simulink model "model1"  (R2024a)
settings: Solver=ode23t  StartTime=0.0  StopTime=finalatt{end,1}  MaxStep=0.1  RelTol=1e-3
undefined symbols (not defined in the file): finalatt, FrontAxle, FrontGear, MassWheel, NewData, RadiusWheel, RearAxle, RearGear, SlipAngle, TrackData, VehicleMass
libraries: fl_lib x16, batt_lib x13, nesl_utility x11, sdl_lib x7, ee_lib x2, simulink x1
(part 2 of 2)

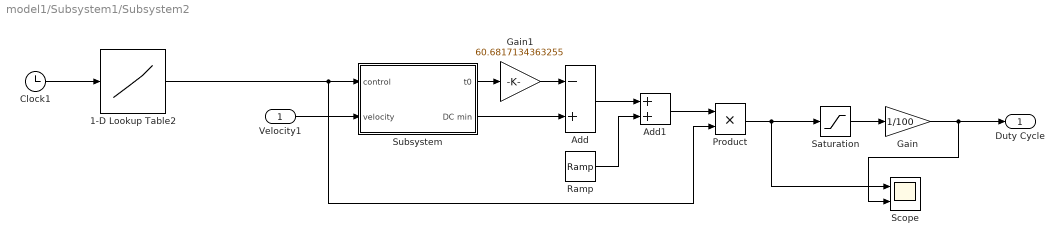
== system model1/Subsystem1/Subsystem2 ==
  Velocity1 : Inport
  1-D Lookup Table2 : Lookup_n-D  NumberOfTableDimensions=1  BreakpointsForDimension1=finalatt{:,1}  Table=finalatt{:,3}  InterpMethod=Flat  InternalRulePriority=Speed  RndMeth=Simplest
  Add : Sum  Inputs=-+
  Add1 : Sum
  Clock1 : Clock
      settings: Decimation=1000
  Gain : Gain  Gain=1/100
  Gain1 : Gain  Gain=60.6817134363255
  Product : Product
  Ramp : simulink/Sources/Ramp  slope=60.6817134363255  start=0  InitialOutput=0
  Saturation : Saturate  UpperLimit=95  LowerLimit=0
  Scope : Scope  NumInputPorts=2
  Subsystem : Subsystem
  Duty Cycle : Outport
  wires:
  Clock1/1 -> 1-D Lookup Table2/1
  Product/1 -> Scope/1, Saturation/1
  Ramp/1 -> Add1/2
  Add1/1 -> Product/1
  Gain1/1 -> Add/1
  Velocity1/1 -> Subsystem/2(velocity)
  Add/1 -> Add1/1
  1-D Lookup Table2/1 -> Product/2, Subsystem/1(control)
  Subsystem/2(DC min) -> Add/2
  Subsystem/1(t0) -> Gain1/1
  Gain/1 -> Scope/2, Duty Cycle/1
  Saturation/1 -> Gain/1

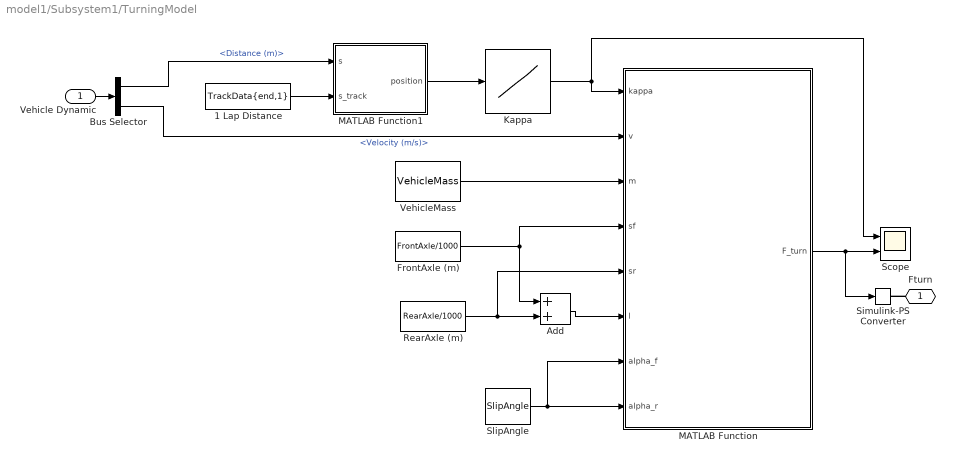
== system model1/Subsystem1/TurningModel ==
  Vehicle Dynamic : Inport
  1 Lap Distance : Constant  Value=TrackData{end,1}
  Add : Sum
  Bus Selector : BusSelector  OutputSignals=Distance (m),Velocity (m/s)
  FrontAxle (m) : Constant  Value=FrontAxle/1000
  Kappa : Lookup_n-D  NumberOfTableDimensions=1  BreakpointsForDimension1=TrackData{:,1}  Table=TrackData{:,4}  InternalRulePriority=Speed  RndMeth=Simplest
  MATLAB Function : MATLAB Function  TreatAsAtomicUnit=on
  MATLAB Function1 : MATLAB Function  TreatAsAtomicUnit=on
  RearAxle (m) : Constant  Value=RearAxle/1000
  Scope : Scope  NumInputPorts=2
  Simulink-PS Converter : nesl_utility/Simulink-PS Converter  PhysicalDomain=network_engine_domain  SubClassName=ps_input  LeftPortType=input  RightPortType=output  PseudoPeriodic=off  Frequencies=[]  NoiseDistribution=none  NoiseParameters=[]  Unit=N  AffineConversion=off  FilteringAndDerivatives=provide  SimscapeFilterOrder=1  InputFilterTimeConstant=0.001  UdotUserProvided=0
  SlipAngle : Constant  Value=SlipAngle
  VehicleMass : Constant  Value=VehicleMass
  Fturn : PMIOPort  Side=Left
  wires:
  VehicleMass/1 -> MATLAB Function/3(m)
  1 Lap Distance/1 -> MATLAB Function1/2(s_track)
  Kappa/1 -> Scope/1, MATLAB Function/1(kappa)
  RearAxle (m)/1 -> MATLAB Function/5(sr), Add/2
  FrontAxle (m)/1 -> MATLAB Function/4(sf), Add/1
  Bus Selector/1 -> MATLAB Function1/1(s)  "<Distance (m)>"
  MATLAB Function1/1(position) -> Kappa/1
  SlipAngle/1 -> MATLAB Function/7(alpha_f), MATLAB Function/8(alpha_r)
  MATLAB Function/1(F_turn) -> Simulink-PS Converter/1, Scope/2
  Vehicle Dynamic/1 -> Bus Selector/1
  Bus Selector/2 -> MATLAB Function/2(v)  "<Velocity (m/s)>"
  Add/1 -> MATLAB Function/6(l)
  connections:
  Fturn/RConn1 -- Simulink-PS Converter/RConn1

== system model1/Subsystem1/VehicleModel ==
  Ideal Force Source : fl_lib/Mechanical/Mechanical Sources/Ideal Force Source
  Mechanical Translational Reference : fl_lib/Mechanical/Translational Elements/Mechanical Translational Reference
  PS Gain : fl_lib/Physical Signals/Functions/PS Gain  gain=0.5
  PS Terminator3 : fl_lib/Physical Signals/Sinks/PS Terminator
  TireModel : Subsystem
      settings: PortSchema="{\"entries\":[{\"content\":{\"sides\":[{\"content\":{\"connectorIds\":[\"LConn1\",\"LConn2\"]},\"type\":\"ConnectorPlacement.EquallySpacedRectSide\",\"uuid\":\"ad88246c-79e4-4500-822e-5fea39c5896c\"},{\"content\":{\"connectorIds\":[\"Out1\"],\"side\":\"RIGHT\"},\"type\":\"ConnectorPlacement.EquallySpacedRectSide\",\"uuid\":\"913d52ca-54a5-4560-b3df-e1f57975974a\"},{\"content\":{\"connectorIds\":[\"LConn3\",\"LConn4\",\"LConn5\"],\"side\":\"TOP\"},\"type\":\"ConnectorPlacement.EquallySpacedRectSide\",\"uuid\":\"5900099e-62c2-49ce-8123-88bd27d24a29\"}]},\"type\":\"ConnectorPlacement.EquallySpacedConnector\",\"uuid\":\"881a997e-2d63-4bf2-b975-40b530568104\"}],\"packageUris\":[\"http://schema.mathworks.com/mf0/Connector/R2020b\"],\"version\":\"1.0\"}"
  Vehicle Body : sdl_lib/Tires & Vehicles/Vehicle Body  mass=VehicleMass kg  n_w=1  x_f=FrontAxle mm  x_r=RearAxle mm  y_c=GroundClearance mm  mass_var=simscape.enum.onoff.off  g=9.81 m/s^2  liftoff_warning=simscape.enum.onoff.off  area=FrontArea m^2  Cd=CD  rho=1.18 kg/m^3  model_pitch=simscape.enum.onoff.off  inertia=4000 kg*m^2  suspension_model=sdl.enum.linearTLU.linear  k_f=1e4 N/m  b_f=1e4 N*s/m  k_r=1e4 N/m  b_r=1e4 N*s/m  k_f_TLU=[-2000, -1000, 0, 1000, 2000] N  x_f_TLU=[-.4, -.2, 0, .2, .4] m  b_f_TLU=[-200, -100, 0, 100, 200] N  v_f_TLU=[-4, -2, 0, 2, 4] m/s  k_r_TLU=[-2000, -1000, 0, 1000, 2000] N  x_r_TLU=[-.4, -.2, 0, .2, .4] m  b_r_TLU=[-200, -100, 0, 100, 200] N  v_r_TLU=[-4, -2, 0, 2, 4] m/s  interp_method=simscape.enum.interpolation.linear  extrap_method=simscape.enum.extrapolation.linear  model_hardstop=simscape.enum.onoff.off  upper_bound_f=.25 m  lower_bound_f=-.25 m  stop_k_f=1e6 N/m  stop_b_f=150 N*s/m  upper_bound_r=.25 m  lower_bound_r=-.25 m  stop_k_r=1e6 N/m  stop_b_r=150 N*s/m  initial_pitch=0 rad  initial_pitch_rate=0 rad/s  v_specify=off  v_priority=High  v=0 m/s  v_nominal_specify=off  v_nominal_value=1  v_nominal_unit=m/s
  FromClutch : PMIOPort  Side=Left
  Fturn : PMIOPort  Port=2  Side=Right
  VehicleDynamic : Outport
  wires:
  TireModel/1(VehicleDynamic) -> VehicleDynamic/1
  connections:
  TireModel/LConn2 -- FromClutch/RConn1
  Vehicle Body/RConn1 -- TireModel/LConn3
  Ideal Force Source/LConn1 -- Mechanical Translational Reference/LConn1
  Ideal Force Source/RConn2 -- TireModel/LConn1 -- Vehicle Body/LConn1
  Fturn/RConn1 -- Ideal Force Source/RConn1
  PS Gain/LConn1 -- Vehicle Body/RConn2
  PS Gain/RConn1 -- TireModel/LConn4
  PS Terminator3/LConn1 -- Vehicle Body/LConn2

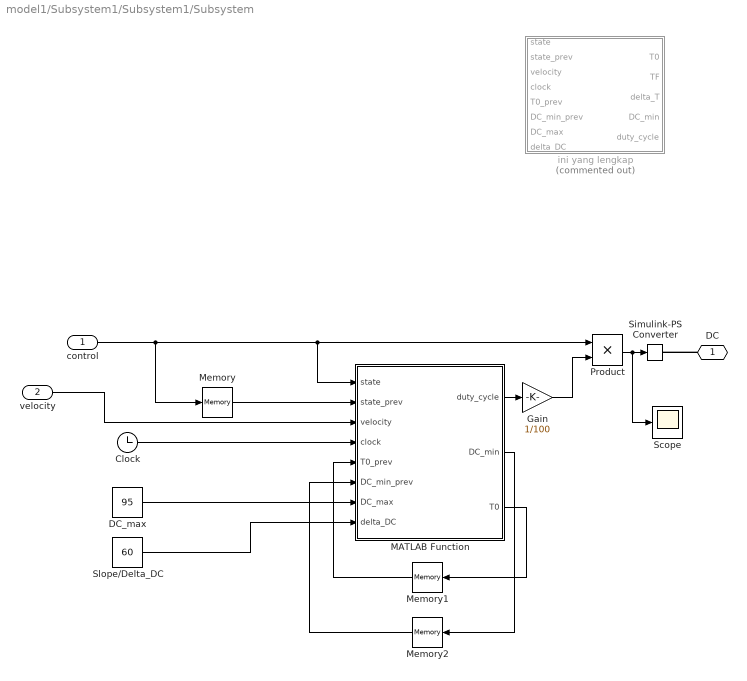
== system model1/Subsystem1/Subsystem1/Subsystem ==
  control : Inport
  velocity : Inport  Port=2
  Clock : Clock
  DC_max : Constant  Value=95
  Gain : Gain  Gain=1/100
  MATLAB Function : MATLAB Function  TreatAsAtomicUnit=on
  Memory : Memory
  Memory1 : Memory
  Memory2 : Memory
  Product : Product
  Scope : Scope
  Simulink-PS Converter : nesl_utility/Simulink-PS Converter  PhysicalDomain=network_engine_domain  SubClassName=ps_input  LeftPortType=input  RightPortType=output  PseudoPeriodic=off  Frequencies=[]  NoiseDistribution=none  NoiseParameters=[]  Unit=1  AffineConversion=off  FilteringAndDerivatives=provide  SimscapeFilterOrder=1  InputFilterTimeConstant=0.001  UdotUserProvided=0
  Slope/Delta_DC : Constant  Value=60
  ini yang lengkap : MATLAB Function  Commented=on  TreatAsAtomicUnit=on
  DC : PMIOPort  Side=Right
  wires:
  Clock/1 -> MATLAB Function/4(clock)
  control/1 -> Memory/1, MATLAB Function/1(state), Product/1
  Memory/1 -> MATLAB Function/2(state_prev)
  velocity/1 -> MATLAB Function/3(velocity)
  DC_max/1 -> MATLAB Function/7(DC_max)
  Slope/Delta_DC/1 -> MATLAB Function/8(delta_DC)
  Product/1 -> Simulink-PS Converter/1, Scope/1
  Memory1/1 -> MATLAB Function/5(T0_prev)
  MATLAB Function/3(T0) -> Memory1/1
  MATLAB Function/2(DC_min) -> Memory2/1
  Memory2/1 -> MATLAB Function/6(DC_min_prev)
  MATLAB Function/1(duty_cycle) -> Gain/1
  Gain/1 -> Product/2
  connections:
  DC/RConn1 -- Simulink-PS Converter/RConn1

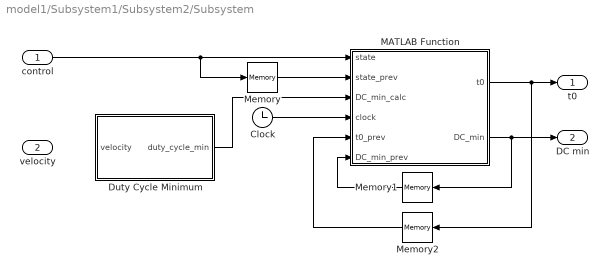
== system model1/Subsystem1/Subsystem2/Subsystem ==
  control : Inport
  velocity : Inport  Port=2
  Clock : Clock
  Duty Cycle Minimum : MATLAB Function  TreatAsAtomicUnit=on
  MATLAB Function : MATLAB Function  TreatAsAtomicUnit=on
  Memory : Memory
  Memory1 : Memory
  Memory2 : Memory
  t0 : Outport
  DC min : Outport  Port=2
  wires:
  MATLAB Function/1(t0) -> Memory2/1, t0/1
  Clock/1 -> MATLAB Function/4(clock)
  control/1 -> Memory/1, MATLAB Function/1(state)
  Memory/1 -> MATLAB Function/2(state_prev)
  MATLAB Function/2(DC_min) -> DC min/1, Memory1/1
  Memory1/1 -> MATLAB Function/6(DC_min_prev)
  Memory2/1 -> MATLAB Function/5(t0_prev)
  Duty Cycle Minimum/1(duty_cycle_min) -> MATLAB Function/3(DC_min_calc)

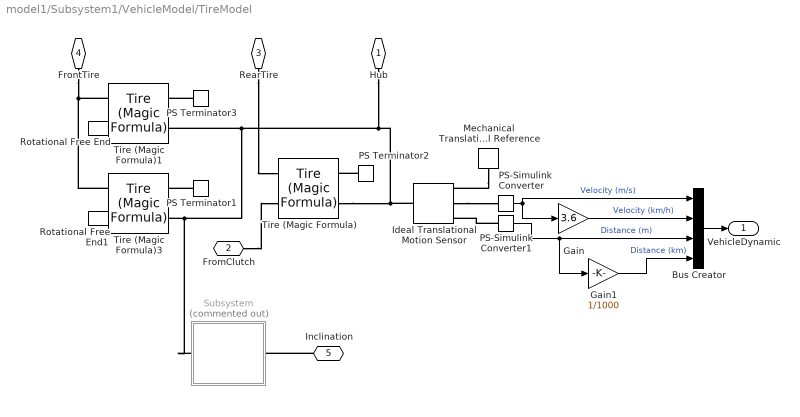
== system model1/Subsystem1/VehicleModel/TireModel ==
  Bus Creator : BusCreator  Inputs=4
  Gain : Gain  Gain=3.6
  Gain1 : Gain  Gain=1/1000
  Ideal Translational Motion Sensor : fl_lib/Mechanical/Mechanical Sensors/Ideal Translational Motion Sensor  reference=foundation.enum.MeasurementReference.difference  acceleration_port=false  velocity_port=true  position_port=true  offset=0 m
  Mechanical Translational Reference : fl_lib/Mechanical/Translational Elements/Mechanical Translational Reference
  PS Terminator1 : fl_lib/Physical Signals/Sinks/PS Terminator
  PS Terminator2 : fl_lib/Physical Signals/Sinks/PS Terminator
  PS Terminator3 : fl_lib/Physical Signals/Sinks/PS Terminator
  PS-Simulink Converter : nesl_utility/PS-Simulink Converter  PhysicalDomain=network_engine_domain  SubClassName=ps_output  LeftPortType=input  RightPortType=output  PseudoPeriodic=off  Frequencies=[]  VectorFormat=1-D array  Unit=m/s  AffineConversion=off
  PS-Simulink Converter1 : nesl_utility/PS-Simulink Converter  PhysicalDomain=network_engine_domain  SubClassName=ps_output  LeftPortType=input  RightPortType=output  PseudoPeriodic=off  Frequencies=[]  VectorFormat=1-D array  Unit=m  AffineConversion=off
  Rotational Free End : fl_lib/Mechanical/Rotational Elements/Rotational Free End  w_specify=off  w_priority=None  w=0 rad/s  w_nominal_specify=off  w_nominal_value=1  w_nominal_unit=rad/s
  Rotational Free End1 : fl_lib/Mechanical/Rotational Elements/Rotational Free End  w_specify=off  w_priority=None  w=0 rad/s  w_nominal_specify=off  w_nominal_value=1  w_nominal_unit=rad/s
  Subsystem : Subsystem  Commented=on
  Tire (Magic Formula) : sdl_lib/Tires & Vehicles/Tire (Magic Formula)  parameterization=sdl.enum.magic_tire_model.peak  F_z1=3000 N  F_x1=3500 N  kappa1=10  B_m=10  C_m=1.9  D_m=1  E_m=0.97  fz0=4000 N  p_Cx=1.685  p_Dx=[1.21, -.037]  p_Ex=[.344, .095, -.02, 0]  p_Kx=[21.51, -.163, .245]  p_Hx=[-.002, .002]  p_Vx=[0, 0]  rolling_radius_model=sdl.enum.RollingRadiusParameterization.Constant  r_e=RadiusWheel m  r_0=0.3 m  breff=8.39  dreff=0.26  freff=0.074  q_re0=0.99  q_v1=0.008  longvl=17 m/s  cz=5e5 N/m  model_resistance=true  resistance_model=sdl.enum.rollingResistanceParameterization.constant  coeff=CRR  p_tire=250e3 Pa  alpha=-0.003  beta=0.97  coeff_a=84e-4  coeff_b=6.2e-4 s/m  coeff_c=1.6e-4 s^2/m^2  p_tire0=240e3 Pa  fz0_resistance=4000 N  vH0=16 m/s  q_Sy=[.0082, 0, .0014, .001, 0, 0, 1.08, -.5]  v_thr=0.001 m/s  enable_scaling_coefficients=false  lfzO=1  lcx=1  lmux=1  lex=1  lkx=1  lhx=1  lvx=1  lmy=1  model_compliance=sdl.enum.compliance.off  stiffness=1e6 N/m  damping=1000 N*s/m  model_inertia=sdl.enum.model_inertia.on  inertia=MassWheel*RadiusWheel^2 kg*m^2  initial_velocity=0 rad/s  vxlow=1 m/s  v_tr_thr=0.1 m/s  kpumin=-1.5  kpumax=1.5
  Tire (Magic Formula)1 : sdl_lib/Tires & Vehicles/Tire (Magic Formula)  parameterization=sdl.enum.magic_tire_model.peak  F_z1=3000 N  F_x1=3500 N  kappa1=10  B_m=10  C_m=1.9  D_m=1  E_m=0.97  fz0=4000 N  p_Cx=1.685  p_Dx=[1.21, -.037]  p_Ex=[.344, .095, -.02, 0]  p_Kx=[21.51, -.163, .245]  p_Hx=[-.002, .002]  p_Vx=[0, 0]  rolling_radius_model=sdl.enum.RollingRadiusParameterization.Constant  r_e=RadiusWheel m  r_0=0.3 m  breff=8.39  dreff=0.26  freff=0.074  q_re0=0.99  q_v1=0.008  longvl=17 m/s  cz=5e5 N/m  model_resistance=true  resistance_model=sdl.enum.rollingResistanceParameterization.constant  coeff=CRR  p_tire=250e3 Pa  alpha=-0.003  beta=0.97  coeff_a=84e-4  coeff_b=6.2e-4 s/m  coeff_c=1.6e-4 s^2/m^2  p_tire0=240e3 Pa  fz0_resistance=4000 N  vH0=16 m/s  q_Sy=[.0082, 0, .0014, .001, 0, 0, 1.08, -.5]  v_thr=0.001 m/s  enable_scaling_coefficients=false  lfzO=1  lcx=1  lmux=1  lex=1  lkx=1  lhx=1  lvx=1  lmy=1  model_compliance=sdl.enum.compliance.off  stiffness=1e6 N/m  damping=1000 N*s/m  model_inertia=sdl.enum.model_inertia.on  inertia=MassWheel*RadiusWheel^2 kg*m^2  initial_velocity=0 rad/s  vxlow=1 m/s  v_tr_thr=0.1 m/s  kpumin=-1.5  kpumax=1.5
  Tire (Magic Formula)3 : sdl_lib/Tires & Vehicles/Tire (Magic Formula)  parameterization=sdl.enum.magic_tire_model.peak  F_z1=3000 N  F_x1=3500 N  kappa1=10  B_m=10  C_m=1.9  D_m=1  E_m=0.97  fz0=4000 N  p_Cx=1.685  p_Dx=[1.21, -.037]  p_Ex=[.344, .095, -.02, 0]  p_Kx=[21.51, -.163, .245]  p_Hx=[-.002, .002]  p_Vx=[0, 0]  rolling_radius_model=sdl.enum.RollingRadiusParameterization.Constant  r_e=RadiusWheel m  r_0=0.3 m  breff=8.39  dreff=0.26  freff=0.074  q_re0=0.99  q_v1=0.008  longvl=17 m/s  cz=5e5 N/m  model_resistance=true  resistance_model=sdl.enum.rollingResistanceParameterization.constant  coeff=CRR  p_tire=250e3 Pa  alpha=-0.003  beta=0.97  coeff_a=84e-4  coeff_b=6.2e-4 s/m  coeff_c=1.6e-4 s^2/m^2  p_tire0=240e3 Pa  fz0_resistance=4000 N  vH0=16 m/s  q_Sy=[.0082, 0, .0014, .001, 0, 0, 1.08, -.5]  v_thr=0.001 m/s  enable_scaling_coefficients=false  lfzO=1  lcx=1  lmux=1  lex=1  lkx=1  lhx=1  lvx=1  lmy=1  model_compliance=sdl.enum.compliance.off  stiffness=1e6 N/m  damping=1000 N*s/m  model_inertia=sdl.enum.model_inertia.on  inertia=MassWheel*RadiusWheel^2 kg*m^2  initial_velocity=0 rad/s  vxlow=1 m/s  v_tr_thr=0.1 m/s  kpumin=-1.5  kpumax=1.5
  Hub : PMIOPort  Side=Left
  FromClutch : PMIOPort  Port=2  Side=Left
  RearTire : PMIOPort  Port=3  Side=Left
  FrontTire : PMIOPort  Port=4  Side=Left
  Inclination : PMIOPort  Port=5  Side=Left
  VehicleDynamic : Outport
  wires:
  PS-Simulink Converter1/1 -> Gain1/1, Bus Creator/3  "Distance (m)"
  PS-Simulink Converter/1 -> Bus Creator/1, Gain/1  "Velocity (m/s)"
  Gain/1 -> Bus Creator/2  "Velocity (km/h)"
  Bus Creator/1 -> VehicleDynamic/1
  Gain1/1 -> Bus Creator/4  "Distance (km)"
  connections:
  PS Terminator3/LConn1 -- Tire (Magic Formula)1/RConn1
  FrontTire/RConn1 -- Tire (Magic Formula)1/LConn1 -- Tire (Magic Formula)3/LConn1
  Tire (Magic Formula)/RConn2 -- Ideal Translational Motion Sensor/LConn1 -- Hub/RConn1 -- Tire (Magic Formula)1/RConn2 -- Subsystem/RConn1 -- Tire (Magic Formula)3/RConn2
  Tire (Magic Formula)1/LConn2 -- Rotational Free End/LConn1
  Tire (Magic Formula)3/LConn2 -- Rotational Free End1/LConn1
  PS Terminator1/LConn1 -- Tire (Magic Formula)3/RConn1
  RearTire/RConn1 -- Tire (Magic Formula)/LConn1
  PS Terminator2/LConn1 -- Tire (Magic Formula)/RConn1
  FromClutch/RConn1 -- Tire (Magic Formula)/LConn2
  Mechanical Translational Reference/LConn1 -- Ideal Translational Motion Sensor/RConn1
  PS-Simulink Converter1/LConn1 -- Ideal Translational Motion Sensor/RConn3
  Ideal Translational Motion Sensor/RConn2 -- PS-Simulink Converter/LConn1
  Inclination/RConn1 -- Subsystem/LConn1

== system model1/Subsystem1/VehicleModel/TireModel/Subsystem ==
  PS-Simulink Converter2 : nesl_utility/PS-Simulink Converter  Commented=on  PhysicalDomain=network_engine_domain  SubClassName=ps_output  LeftPortType=input  RightPortType=output  PseudoPeriodic=off  Frequencies=[]  VectorFormat=inherit  Unit=inherit  AffineConversion=off
  Road Profile : sdl_lib/Tires & Vehicles/Road Profile  Commented=on  x_f=FrontAxle mm  x_r=RearAxle mm  x_height_vector=TrackData{:,1} m  height_vector=TrackData{:,6} m  friction_output=sdl.enum.tire_friction_model.none  x_friction_vector=[-10, 2, 2.1, 6, 6.1, 10] m  MF_M_matrix=[10, 2, 1, 1; 10, 2, 1, 1; 8, 3, 1, 1; 8, 3, 1, 1; 9, 4, 1, 1; 9, 4, 1, 1]  MR_M_matrix=[10, 2, 1, 1; 10, 2, 1, 1; 8, 3, 1, 1; 8, 3, 1, 1; 9, 4, 1, 1; 9, 4, 1, 1]  MF_F_matrix=[.9, .7; .9, .7; .7, .5; .7, .5; .8, .6; .8, .6]  MR_F_matrix=[.9, .7; .9, .7; .7, .5; .7, .5; .8, .6; .8, .6]  x_specify=off  x_priority=High  x=0 m  x_nominal_specify=off  x_nominal_value=1  x_nominal_unit=m
      settings: InternalSimscapePortConfiguration="{\"Bottom\":[],\"Left\":[],\"Right\":[{\"id\":\"H\",\"label\":\"H\",\"type\":\"foundation.mechanical.translational.translational\"},{\"id\":\"beta\",\"label\":\"beta\",\"type\":\"output\"}],\"Top\":[]}"
  Scope : Scope  Commented=on
  Conn1 : PMIOPort  Side=Right
  Inclination : PMIOPort  Port=2  Side=Left
  wires:
  PS-Simulink Converter2/1 -> Scope/1
  connections:
  PS-Simulink Converter2/LConn1 -- Inclination/RConn1 -- Road Profile/RConn2
  Road Profile/RConn1 -- Conn1/RConn1

== matlab function model1/Subsystem1/TurningModel/MATLAB Function1 ==
  data: s input; position output; s_track input
function position = fcn(s, s_track)

if s <= s_track
    position = ceil(s);
else
    position = ceil(s - (ceil(s/s_track) - 1)*s_track);
end

== matlab function model1/Subsystem1/TurningModel/MATLAB Function ==
  data: kappa input; F_turn output; v input; m input; sf input; sr input; l input; alpha_f input; alpha_r input
function F_turn = calculate_turn_resistance(kappa, v, m,sf,sr,l,alpha_f,alpha_r)
% Calculate turn resistance force
% Inputs:
%   kappa - curvature (rad/m)
%   v - velocity (m/s)
%   m - mass (kg)
%   sf - CoM to front axle (m)
%   sr - CoM to rear axle (m)
%   l - wheelbase (m)
%   alpha_f - front slip angle (rad)
%   alpha_r - rear slip angle (rad)

% Avoid division by zero

if abs(kappa) < 1e-6
    R_turn = 1e6;  % Very large radius for straight line
else
    R_turn = 1 / kappa;
end

% Calculate turn resistance
mv2 = m * v^2;
slip_term = sf * alpha_f + sr * alpha_r;
F_turn = (mv2 / (R_turn * l)) * slip_term;

% Ensure non-negative force
F_turn = abs(F_turn);
end

== matlab function model1/Subsystem1/Subsystem1/Subsystem/MATLAB Function ==
  data: state input; duty_cycle output; state_prev input; velocity input; clock input; T0_prev input; DC_min_prev input; DC_max input; delta_DC input; DC_min output; T0 output
function [duty_cycle,DC_min, T0] = fcn(state, state_prev, velocity, clock, T0_prev, DC_min_prev, DC_max, delta_DC)
    % Input:
    % state: current state (0/1)
    % state_prev: previous state
    % velocity: current velocity (m/s)
    % clock: current time
    % T0_prev: previous start time value
    % DC_min_prev: previous DC_min value
    % DC_max: maximum duty cycle (95)
    % delta_DC: ramp slope (60 %/s)
    
    % Output:
    % duty_cycle: current duty cycle output
    
    % 1. Calculate DC_min from velocity
    DC_min_calc = velocity * 95 / 32;
    
    % 2. State logic to determine T0 and DC_min
    if state_prev == 0 && state == 1
        % OFF → ON transition: Start new ramp
        T0 = clock;           % Start time is now
        DC_min = DC_min_calc; % Use new DC_min
        
    elseif state_prev == 1 && state == 1
        % ON continues: Keep previous values
        T0 = T0_prev;         % Keep same start time
        DC_min = DC_min_prev; % Keep same DC_min
        
    else
        % OFF state or ON→OFF transition
        T0 = clock;           % Reset start time
        DC_min = DC_min_calc; % Use current DC_min
    end
    
    % 3. Calculate delta_T (elapsed time since ramp start)
    delta_T = clock - T0;
    if delta_T < 0
        delta_T = 0;  % Safety check
    end
    
    % 4. Calculate duty cycle based on state
    if state == 1
        % ON state: Ramp calculation
        duty_ramp = DC_min + delta_DC * delta_T;
        
        % Apply saturation to DC_max
        if duty_ramp > DC_max
            duty_cycle = DC_max;
        else
            duty_cycle = duty_ramp;
        end
    else
        % OFF state: Direct to DC_min
        duty_cycle = DC_min;
    end
    
    % 5. Final saturation (0% to DC_max)
    if duty_cycle < 0
        duty_cycle = 0;
    elseif duty_cycle > DC_max
        duty_cycle = DC_max;
    end
end

== matlab function model1/Subsystem1/Subsystem1/Subsystem/ini yang lengkap ==
  data: T0 output; TF output; delta_T output; DC_min output; state input; state_prev input; velocity input; clock input; T0_prev input; DC_min_prev input; DC_max input; duty_cycle output; delta_DC input
function [T0, TF, delta_T, DC_min, duty_cycle] = fcn(state, state_prev, velocity, clock, T0_prev, DC_min_prev, DC_max, delta_DC)
    % Input:
    % state: current state (0/1)
    % state_prev: previous state
    % velocity: current velocity (m/s)
    % clock: current time (TF)
    % T0_prev: previous T0 value
    % DC_min_prev: previous DC_min value
    % DC_max: maximum duty cycle (95)
    % delta_DC: ramp slope (60 %/s)
    
    % Output:
    % T0: start time of current ramp
    % TF: current time (same as input clock)
    % delta_T: elapsed time since ramp start (TF - T0)
    % DC_min: current minimum duty cycle
    % duty_cycle: current duty cycle output
    
    % 1. Calculate DC_min from velocity
    DC_min_calc = velocity * 95 / 32;
    
    % 2. State logic to determine T0 and DC_min
    if state_prev == 0 && state == 1
        % OFF → ON transition: Start new ramp
        T0 = clock;           % Start time is now
        DC_min = DC_min_calc; % Use new DC_min
        
    elseif state_prev == 1 && state == 1
        % ON continues: Keep previous values
        T0 = T0_prev;         % Keep same start time
        DC_min = DC_min_prev; % Keep same DC_min
        
    else
        % OFF state or ON→OFF transition
        T0 = clock;           % Reset start time
        DC_min = DC_min_calc; % Use current DC_min
    end
    
    % 3. TF is always the current time
    TF = clock;
    
    % 4. Calculate delta_T (elapsed time since ramp start)
    delta_T = TF - T0;
    if delta_T < 0
        delta_T = 0;  % Safety check
    end
    
    % 5. Calculate duty cycle based on state
    if state == 1
        % ON state: Ramp calculation
        duty_ramp = DC_min + delta_DC * delta_T;
        
        % Apply saturation to DC_max
        if duty_ramp > DC_max
            duty_cycle = DC_max;
        else
            duty_cycle = duty_ramp;
        end
    else
        % OFF state: Direct to DC_min
        duty_cycle = DC_min;
    end
    
    % 6. Final saturation (0% to DC_max)
    if duty_cycle < 0
        duty_cycle = 0;
    elseif duty_cycle > DC_max
        duty_cycle = DC_max;
    end
    
    % 7. Display for debugging (optional)
    % fprintf('TF=%.1f, T0=%.1f, ΔT=%.1f, State=%d, DC_min=%.2f, Duty=%.2f\n',...
    %         TF, T0, delta_T, state, DC_min, duty_cycle);
end

== matlab function model1/Subsystem1/Inclination Model/MATLAB Function1 ==
  data: s input; position output; s_track input
function position = fcn(s, s_track)

if s <= s_track
    position = ceil(s);
else
    position = ceil(s - (ceil(s/s_track) - 1)*s_track);
end

== matlab function model1/Subsystem1/Subsystem2/Subsystem/Duty Cycle Minimum ==
  data: velocity input; duty_cycle_min output
function duty_cycle_min = fcn(velocity)

duty_cycle_min = (95/32)*velocity;

== matlab function model1/Subsystem1/Subsystem2/Subsystem/MATLAB Function ==
  data: state input; t0 output; state_prev input; DC_min_calc input; clock input; t0_prev input; DC_min_prev input; DC_min output
function [t0, DC_min] = fcn(state, state_prev, DC_min_calc, clock, t0_prev, DC_min_prev)

if state_prev==0 && state==1
    t0 = clock;
    DC_min = DC_min_calc;
    
elseif state_prev==1 && state==1
    t0 = t0_prev;
    DC_min = DC_min_prev;
else
    t0 = clock;
    DC_min = DC_min_calc;
end
